simulink model "simulacionMotorDC"  (R2014a)
settings: Solver=ode45  StartTime=0.0  StopTime=10.0  RelTol=1e-3
settings Model: Creator=PedroBarquin  LastModifiedBy=PedroBarquin

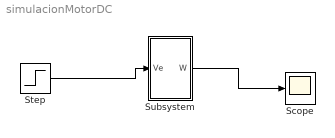
== system simulacionMotorDC ==
  Scope : Scope
  Step : Step  SampleTime=0
  Subsystem : Subsystem  mask{A=1, b=1, omega_0=0}
  wires:
  Step/1 -> Subsystem/1(Ve)
  Subsystem/1("W ") -> Scope/1

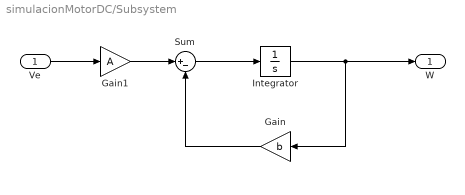
== system simulacionMotorDC/Subsystem ==
  Ve : Inport
  Gain : Gain  Gain=b
  Gain1 : Gain  Gain=A
  Integrator : Integrator  InitialCondition=omega_0
  Sum : Sum  Inputs=|+-
  "W " : Outport
  wires:
  Gain1/1 -> Sum/1
  Sum/1 -> Integrator/1
  Ve/1 -> Gain1/1
  Gain/1 -> Sum/2
  Integrator/1 -> "W "/1, Gain/1
